simulink model "sampleModel7126_pp"  (R2018a)
settings: Solver=VariableStepAuto  StartTime=0.0  StopTime=10.0  RelTol=1e-3
undefined symbols (not defined in the file or in its folder): DiscIntNeverNeededParam
libraries: simulink x367
(part 3 of 8)

== system sampleModel7126_pp/cfblk260 ==
  cfblk1 : Inport
  cfblk9 : Inport  Port=2
  Action Port : ActionPort  ActionType=else
  cfblk13 : Delay
  cfblk3 : simulink/Discrete/Transfer Fcn Real Zero  ZeroZ=0.75  ICPrevInput=0.0  DoSatur=off
      settings: SourceProductName=Simulink  SourceProductBaseCode=SL
  cfblk4 : simulink/Continuous/PID Controller  Controller=PID  TimeDomain=Discrete-time  SampleTime=-1  IntegratorMethod=Forward Euler  FilterMethod=Forward Euler  Form=Parallel  UseFilter=on  ControllerParametersSource=internal  P=1  I=1  D=0  N=100  InitialConditionSource=internal  InitialConditionForIntegrator=0  InitialConditionForFilter=0  ExternalReset=none  LimitOutput=off  UpperSaturationLimit=inf  LowerSaturationLimit=-inf  LinearizeAsGain=off  AntiWindupMode=none  Kb=1  TrackingMode=off  Kt=1  PParamMin=[]  PParamMax=[]  IParamMin=[]  IParamMax=[]  DParamMin=[]  DParamMax=[]  NParamMin=[]  NParamMax=[]  KbParamMin=[]  KbParamMax=[]  KtParamMin=[]  KtParamMax=[]  POutMin=[]  POutMax=[]  IOutMin=[]  IOutMax=[]  DOutMin=[]  DOutMax=[]  NOutMin=[]  NOutMax=[]  KbOutMin=[]  KbOutMax=[]  KtOutMin=[]  KtOutMax=[]  IntegratorOutMin=[]  IntegratorOutMax=[]  FilterOutMin=[]  FilterOutMax=[]  SumOutMin=[]  SumOutMax=[]  SumI1OutMin=[]  SumI1OutMax=[]  SumI2OutMin=[]  SumI2OutMax=[]  SumI3OutMin=[]  SumI3OutMax=[]  SumDOutMin=[]  SumDOutMax=[]  SaturationOutMin=[]  SaturationOutMax=[]  IntegratorContinuousStateAttributes=''  IntegratorStateMustResolveToSignalObject=off  IntegratorRTWStateStorageClass=Auto  FilterContinuousStateAttributes=''  FilterStateMustResolveToSignalObject=off  FilterRTWStateStorageClass=Auto  DifferentiatorICPrevScaledInput=0  DifferentiatorOutMin=[]  DifferentiatorOutMax=[]  FilterDiffOutCoefMin=[]  FilterDiffOutCoefMax=[]  SumDenOutMin=[]  SumDenOutMax=[]  SumNumOutMin=[]  SumNumOutMax=[]  ReciprocalOutMin=[]  ReciprocalOutMax=[]  DivideOutMin=[]  DivideOutMax=[]  TunerSelectOption=Transfer Function Based (PID Tuner App)
  cfblk5 : DiscreteIntegrator  SampleTime=-1  OutDataTypeStr=double  ICPrevOutput=DiscIntNeverNeededParam  ICPrevScaledInput=DiscIntNeverNeededParam
  cfblk6 : Delay
  cfblk7 : Delay  DelayLengthSource=Input port
      settings: InputPortMap=u0,p1
  cfblk8 : simulink/Discrete/Transfer Fcn Lead or Lag  PoleZ=0.95  ZeroZ=0.75  ICPrevOutput=0.0  ICPrevInput=0.0  DoSatur=off
      settings: SourceProductName=Simulink  SourceProductBaseCode=SL
  cyemi_{449..456} (8 alike) : DataTypeConversion  OutDataTypeStr=double
  cfblk2 : Outport
  cfblk10 : Outport  Port=2
  cfblk11 : Outport  Port=3
  cfblk12 : Outport  Port=4
  wires:
  cfblk8/1 -> cfblk10/1
  cfblk4/1 -> cfblk12/1, cyemi_453/1
  cfblk3/1 -> cyemi_451/1, cyemi_452/1
  cfblk9/1 -> cfblk11/1, cfblk2/1
  cyemi_449/1 -> cfblk13/1
  cfblk5/1 -> cyemi_449/1
  cyemi_450/1 -> cfblk3/1
  cfblk13/1 -> cyemi_450/1
  cyemi_451/1 -> cfblk4/1
  cyemi_452/1 -> cfblk5/1
  cyemi_453/1 -> cfblk6/1
  cyemi_454/1 -> cfblk7/1
  cfblk6/1 -> cyemi_454/1
  cyemi_455/1 -> cfblk7/2
  cfblk1/1 -> cyemi_455/1
  cyemi_456/1 -> cfblk8/1
  cfblk7/1 -> cyemi_456/1

== system sampleModel7126_pp/cfblk261 ==
  cfblk1 : Inport
  Action Port : ActionPort  ActionType=then
  cfblk10 : simulink/Discrete/Difference  ICPrevInput=0.0  OutMin=[]  OutMax=[]  OutDataTypeStr=double  OutputDataTypeScalingMode=double  OutDataType=fixdt(1, 16)  OutScaling=2^-10  DoSatur=off
  cfblk11 : If  SampleTime=1
  cfblk13 : Subsystem  TreatAsAtomicUnit=on
  cfblk14 : Subsystem  TreatAsAtomicUnit=on
  cfblk15 : Delay
  cfblk16 : Delay
  cfblk17 : Delay
  cfblk3 : simulink/Discrete/Difference  ICPrevInput=0.0  OutMin=[]  OutMax=[]  OutDataTypeStr=double  OutputDataTypeScalingMode=double  OutDataType=fixdt(1, 16)  OutScaling=2^-10  DoSatur=off
  cfblk4 : DiscreteFilter
  cfblk5 : DiscreteTransferFcn
  cfblk6 : simulink/Continuous/PID Controller (2DOF)  Controller=PID  TimeDomain=Discrete-time  SampleTime=-1  IntegratorMethod=Forward Euler  FilterMethod=Forward Euler  Form=Parallel  UseFilter=on  ControllerParametersSource=internal  P=1  I=1  D=0  N=100  b=1  c=1  InitialConditionSource=internal  InitialConditionForIntegrator=0  InitialConditionForFilter=0  ExternalReset=none  LimitOutput=off  UpperSaturationLimit=inf  LowerSaturationLimit=-inf  LinearizeAsGain=off  AntiWindupMode=none  Kb=1  TrackingMode=off  Kt=1  PParamMin=[]  PParamMax=[]  IParamMin=[]  IParamMax=[]  DParamMin=[]  DParamMax=[]  NParamMin=[]  NParamMax=[]  bParamMin=[]  bParamMax=[]  cParamMin=[]  cParamMax=[]  KbParamMin=[]  KbParamMax=[]  KtParamMin=[]  KtParamMax=[]  POutMin=[]  POutMax=[]  IOutMin=[]  IOutMax=[]  DOutMin=[]  DOutMax=[]  NOutMin=[]  NOutMax=[]  bOutMin=[]  bOutMax=[]  cOutMin=[]  cOutMax=[]  KbOutMin=[]  KbOutMax=[]  KtOutMin=[]  KtOutMax=[]  IntegratorOutMin=[]  IntegratorOutMax=[]  FilterOutMin=[]  FilterOutMax=[]  SumOutMin=[]  SumOutMax=[]  Sum1OutMin=[]  Sum1OutMax=[]  Sum2OutMin=[]  Sum2OutMax=[]  Sum3OutMin=[]  Sum3OutMax=[]  SumI1OutMin=[]  SumI1OutMax=[]  SumI2OutMin=[]  SumI2OutMax=[]  SumI3OutMin=[]  SumI3OutMax=[]  SumDOutMin=[]  SumDOutMax=[]  SaturationOutMin=[]  SaturationOutMax=[]  IntegratorContinuousStateAttributes=''  IntegratorStateMustResolveToSignalObject=off  IntegratorRTWStateStorageClass=Auto  FilterContinuousStateAttributes=''  FilterStateMustResolveToSignalObject=off  FilterRTWStateStorageClass=Auto  DifferentiatorICPrevScaledInput=0  DifferentiatorOutMin=[]  DifferentiatorOutMax=[]  FilterDiffOutCoefMin=[]  FilterDiffOutCoefMax=[]  SumDenOutMin=[]  SumDenOutMax=[]  SumNumOutMin=[]  SumNumOutMax=[]  ReciprocalOutMin=[]  ReciprocalOutMax=[]  DivideOutMin=[]  DivideOutMax=[]  TunerSelectOption=Transfer Function Based (PID Tuner App)
  cfblk7 : Delay  ShowEnablePort=on
      settings: InputPortMap=u0,e6
  cfblk8 : DiscreteZeroPole  Poles=[0 0.5]  Gain=1  SampleTime=-1
  cfblk9 : simulink/Continuous/PID Controller  Controller=PID  TimeDomain=Discrete-time  SampleTime=-1  IntegratorMethod=Forward Euler  FilterMethod=Forward Euler  Form=Parallel  UseFilter=on  ControllerParametersSource=internal  P=1  I=1  D=0  N=100  InitialConditionSource=internal  InitialConditionForIntegrator=0  InitialConditionForFilter=0  ExternalReset=none  LimitOutput=off  UpperSaturationLimit=inf  LowerSaturationLimit=-inf  LinearizeAsGain=off  AntiWindupMode=none  Kb=1  TrackingMode=off  Kt=1  PParamMin=[]  PParamMax=[]  IParamMin=[]  IParamMax=[]  DParamMin=[]  DParamMax=[]  NParamMin=[]  NParamMax=[]  KbParamMin=[]  KbParamMax=[]  KtParamMin=[]  KtParamMax=[]  POutMin=[]  POutMax=[]  IOutMin=[]  IOutMax=[]  DOutMin=[]  DOutMax=[]  NOutMin=[]  NOutMax=[]  KbOutMin=[]  KbOutMax=[]  KtOutMin=[]  KtOutMax=[]  IntegratorOutMin=[]  IntegratorOutMax=[]  FilterOutMin=[]  FilterOutMax=[]  SumOutMin=[]  SumOutMax=[]  SumI1OutMin=[]  SumI1OutMax=[]  SumI2OutMin=[]  SumI2OutMax=[]  SumI3OutMin=[]  SumI3OutMax=[]  SumDOutMin=[]  SumDOutMax=[]  SaturationOutMin=[]  SaturationOutMax=[]  IntegratorContinuousStateAttributes=''  IntegratorStateMustResolveToSignalObject=off  IntegratorRTWStateStorageClass=Auto  FilterContinuousStateAttributes=''  FilterStateMustResolveToSignalObject=off  FilterRTWStateStorageClass=Auto  DifferentiatorICPrevScaledInput=0  DifferentiatorOutMin=[]  DifferentiatorOutMax=[]  FilterDiffOutCoefMin=[]  FilterDiffOutCoefMax=[]  SumDenOutMin=[]  SumDenOutMax=[]  SumNumOutMin=[]  SumNumOutMax=[]  ReciprocalOutMin=[]  ReciprocalOutMax=[]  DivideOutMin=[]  DivideOutMax=[]  TunerSelectOption=Transfer Function Based (PID Tuner App)
  cyemi_{458..460,469..470,473..484} (17 alike) : DataTypeConversion  OutDataTypeStr=double
  cfblk2 : Outport
  cfblk12 : Outport  Port=2
  wires:
  cfblk7/1 -> cyemi_459/1, cyemi_476/1
  cfblk9/1 -> cfblk2/1
  cfblk8/1 -> cyemi_473/1, cyemi_478/1
  cfblk13/1(cfblk2) -> cyemi_470/1, cyemi_479/1
  cfblk14/1(cfblk2) -> cfblk12/1
  cfblk11/1 -> cfblk13/Action
  cfblk11/2 -> cfblk14/Action
  cyemi_458/1 -> cfblk10/1
  cfblk14/3(cfblk7) -> cyemi_458/1
  cyemi_459/1 -> cfblk11/1
  cyemi_460/1 -> cfblk13/1(cfblk1)
  cfblk3/1 -> cyemi_460/1
  cyemi_469/1 -> cfblk14/1(cfblk1)
  cfblk16/1 -> cyemi_469/1
  cyemi_470/1 -> cfblk14/2(cfblk5)
  cyemi_473/1 -> cfblk15/1
  cyemi_474/1 -> cfblk16/1
  cfblk4/1 -> cyemi_474/1
  cyemi_475/1 -> cfblk17/1
  cfblk10/1 -> cyemi_475/1
  cyemi_476/1 -> cfblk3/1
  cyemi_477/1 -> cfblk4/1
  cfblk14/2(cfblk6) -> cyemi_477/1
  cyemi_478/1 -> cfblk5/1
  cyemi_479/1 -> cfblk6/1
  cyemi_480/1 -> cfblk6/2
  cfblk15/1 -> cyemi_480/1
  cyemi_481/1 -> cfblk7/1
  cfblk1/1 -> cyemi_481/1
  cyemi_482/1 -> cfblk7/2
  cfblk17/1 -> cyemi_482/1
  cyemi_483/1 -> cfblk8/1
  cfblk6/1 -> cyemi_483/1
  cyemi_484/1 -> cfblk9/1
  cfblk5/1 -> cyemi_484/1

== system sampleModel7126_pp/cfblk262 ==
  cfblk1 : Inport
  cfblk9 : Inport  Port=2
  Action Port : ActionPort  ActionType=else
  cfblk11 : Delay
  cfblk3 : simulink/Continuous/PID Controller  Controller=PID  TimeDomain=Discrete-time  SampleTime=-1  IntegratorMethod=Forward Euler  FilterMethod=Forward Euler  Form=Parallel  UseFilter=on  ControllerParametersSource=internal  P=1  I=1  D=0  N=100  InitialConditionSource=internal  InitialConditionForIntegrator=0  InitialConditionForFilter=0  ExternalReset=none  LimitOutput=off  UpperSaturationLimit=inf  LowerSaturationLimit=-inf  LinearizeAsGain=off  AntiWindupMode=none  Kb=1  TrackingMode=off  Kt=1  PParamMin=[]  PParamMax=[]  IParamMin=[]  IParamMax=[]  DParamMin=[]  DParamMax=[]  NParamMin=[]  NParamMax=[]  KbParamMin=[]  KbParamMax=[]  KtParamMin=[]  KtParamMax=[]  POutMin=[]  POutMax=[]  IOutMin=[]  IOutMax=[]  DOutMin=[]  DOutMax=[]  NOutMin=[]  NOutMax=[]  KbOutMin=[]  KbOutMax=[]  KtOutMin=[]  KtOutMax=[]  IntegratorOutMin=[]  IntegratorOutMax=[]  FilterOutMin=[]  FilterOutMax=[]  SumOutMin=[]  SumOutMax=[]  SumI1OutMin=[]  SumI1OutMax=[]  SumI2OutMin=[]  SumI2OutMax=[]  SumI3OutMin=[]  SumI3OutMax=[]  SumDOutMin=[]  SumDOutMax=[]  SaturationOutMin=[]  SaturationOutMax=[]  IntegratorContinuousStateAttributes=''  IntegratorStateMustResolveToSignalObject=off  IntegratorRTWStateStorageClass=Auto  FilterContinuousStateAttributes=''  FilterStateMustResolveToSignalObject=off  FilterRTWStateStorageClass=Auto  DifferentiatorICPrevScaledInput=0  DifferentiatorOutMin=[]  DifferentiatorOutMax=[]  FilterDiffOutCoefMin=[]  FilterDiffOutCoefMax=[]  SumDenOutMin=[]  SumDenOutMax=[]  SumNumOutMin=[]  SumNumOutMax=[]  ReciprocalOutMin=[]  ReciprocalOutMax=[]  DivideOutMin=[]  DivideOutMax=[]  TunerSelectOption=Transfer Function Based (PID Tuner App)
  cfblk4 : DiscreteIntegrator  SampleTime=-1  OutDataTypeStr=double  ICPrevOutput=DiscIntNeverNeededParam  ICPrevScaledInput=DiscIntNeverNeededParam
  cfblk5 : Delay  DelayLengthSource=Input port
      settings: InputPortMap=u0,p1
  cfblk6 : simulink/Discrete/Transfer Fcn Real Zero  ZeroZ=0.75  ICPrevInput=0.0  DoSatur=off
      settings: SourceProductName=Simulink  SourceProductBaseCode=SL
  cfblk7 : DiscreteFilter
  cfblk8 : Delay
  cyemi_{487..494} (8 alike) : DataTypeConversion  OutDataTypeStr=double
  cfblk2 : Outport
  cfblk10 : Outport  Port=2
  wires:
  cfblk7/1 -> cfblk2/1
  cfblk9/1 -> cfblk10/1
  cfblk8/1 -> cyemi_487/1, cyemi_488/1
  cyemi_487/1 -> cfblk11/1
  cyemi_488/1 -> cfblk3/1
  cyemi_489/1 -> cfblk4/1
  cfblk1/1 -> cyemi_489/1
  cyemi_490/1 -> cfblk5/1
  cfblk6/1 -> cyemi_490/1
  cyemi_491/1 -> cfblk5/2
  cfblk11/1 -> cyemi_491/1
  cyemi_492/1 -> cfblk6/1
  cfblk4/1 -> cyemi_492/1
  cyemi_493/1 -> cfblk7/1
  cfblk3/1 -> cyemi_493/1
  cyemi_494/1 -> cfblk8/1
  cfblk5/1 -> cyemi_494/1

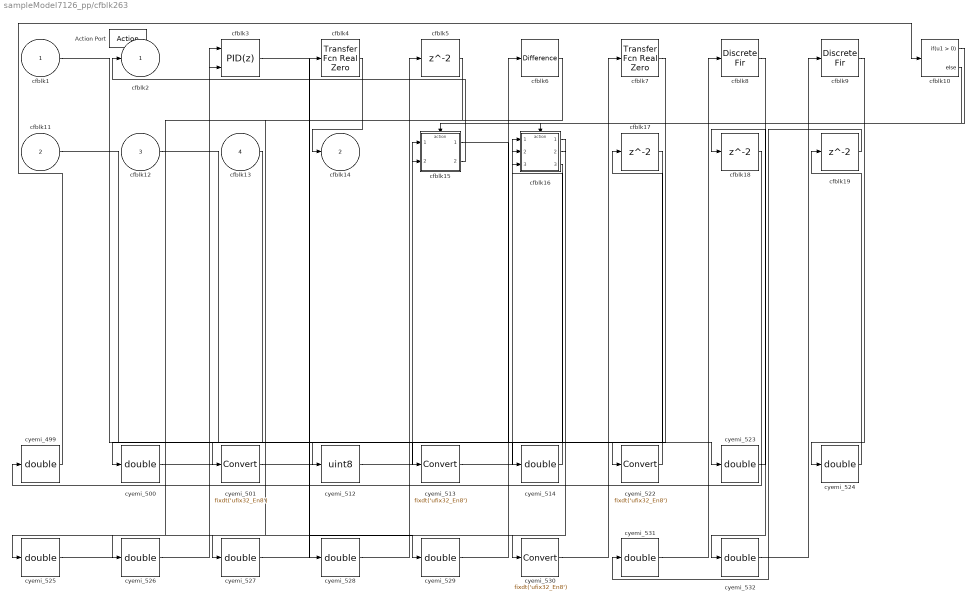
== system sampleModel7126_pp/cfblk263 ==
  cfblk1 : Inport
  cfblk11 : Inport  Port=2
  cfblk12 : Inport  Port=3
  cfblk13 : Inport  Port=4
  Action Port : ActionPort  ActionType=then
  cfblk10 : If  SampleTime=1
  cfblk15 : Subsystem  TreatAsAtomicUnit=on
  cfblk16 : Subsystem  TreatAsAtomicUnit=on
  cfblk{5,17..19} (4 alike) : Delay
  cfblk3 : simulink/Continuous/PID Controller (2DOF)  Controller=PID  TimeDomain=Discrete-time  SampleTime=-1  IntegratorMethod=Forward Euler  FilterMethod=Forward Euler  Form=Parallel  UseFilter=on  ControllerParametersSource=internal  P=1  I=1  D=0  N=100  b=1  c=1  InitialConditionSource=internal  InitialConditionForIntegrator=0  InitialConditionForFilter=0  ExternalReset=none  LimitOutput=off  UpperSaturationLimit=inf  LowerSaturationLimit=-inf  LinearizeAsGain=off  AntiWindupMode=none  Kb=1  TrackingMode=off  Kt=1  PParamMin=[]  PParamMax=[]  IParamMin=[]  IParamMax=[]  DParamMin=[]  DParamMax=[]  NParamMin=[]  NParamMax=[]  bParamMin=[]  bParamMax=[]  cParamMin=[]  cParamMax=[]  KbParamMin=[]  KbParamMax=[]  KtParamMin=[]  KtParamMax=[]  POutMin=[]  POutMax=[]  IOutMin=[]  IOutMax=[]  DOutMin=[]  DOutMax=[]  NOutMin=[]  NOutMax=[]  bOutMin=[]  bOutMax=[]  cOutMin=[]  cOutMax=[]  KbOutMin=[]  KbOutMax=[]  KtOutMin=[]  KtOutMax=[]  IntegratorOutMin=[]  IntegratorOutMax=[]  FilterOutMin=[]  FilterOutMax=[]  SumOutMin=[]  SumOutMax=[]  Sum1OutMin=[]  Sum1OutMax=[]  Sum2OutMin=[]  Sum2OutMax=[]  Sum3OutMin=[]  Sum3OutMax=[]  SumI1OutMin=[]  SumI1OutMax=[]  SumI2OutMin=[]  SumI2OutMax=[]  SumI3OutMin=[]  SumI3OutMax=[]  SumDOutMin=[]  SumDOutMax=[]  SaturationOutMin=[]  SaturationOutMax=[]  IntegratorContinuousStateAttributes=''  IntegratorStateMustResolveToSignalObject=off  IntegratorRTWStateStorageClass=Auto  FilterContinuousStateAttributes=''  FilterStateMustResolveToSignalObject=off  FilterRTWStateStorageClass=Auto  DifferentiatorICPrevScaledInput=0  DifferentiatorOutMin=[]  DifferentiatorOutMax=[]  FilterDiffOutCoefMin=[]  FilterDiffOutCoefMax=[]  SumDenOutMin=[]  SumDenOutMax=[]  SumNumOutMin=[]  SumNumOutMax=[]  ReciprocalOutMin=[]  ReciprocalOutMax=[]  DivideOutMin=[]  DivideOutMax=[]  TunerSelectOption=Transfer Function Based (PID Tuner App)
  cfblk4 : simulink/Discrete/Transfer Fcn Real Zero  ZeroZ=0.75  ICPrevInput=0.0  DoSatur=off
      settings: SourceProductName=Simulink  SourceProductBaseCode=SL
  cfblk6 : simulink/Discrete/Difference  ICPrevInput=0.0  OutMin=[]  OutMax=[]  OutDataTypeStr=double  OutputDataTypeScalingMode=double  OutDataType=fixdt(1, 16)  OutScaling=2^-10  DoSatur=off
  cfblk7 : simulink/Discrete/Transfer Fcn Real Zero  ZeroZ=0.75  ICPrevInput=0.0  DoSatur=off
      settings: SourceProductName=Simulink  SourceProductBaseCode=SL
  cfblk8 : DiscreteFir
  cfblk9 : DiscreteFir
  cyemi_{499..500,514,523..529,531..532} (12 alike) : DataTypeConversion  OutDataTypeStr=double
  cyemi_{501,513,522,530} (4 alike) : DataTypeConversion  OutDataTypeStr=fixdt('ufix32_En8')
  cyemi_512 : DataTypeConversion  OutDataTypeStr=uint8
  cfblk2 : Outport
  cfblk14 : Outport  Port=2
  wires:
  cfblk4/1 -> cfblk14/1
  cfblk15/2(cfblk12) -> cfblk2/1
  cfblk10/1 -> cfblk15/Action
  cfblk10/2 -> cfblk16/Action
  cyemi_499/1 -> cfblk10/1
  cfblk18/1 -> cyemi_499/1
  cyemi_500/1 -> cfblk15/1(cfblk1)
  cfblk13/1 -> cyemi_500/1
  cyemi_501/1 -> cfblk15/2(cfblk11)
  cfblk16/3(cfblk13) -> cyemi_501/1
  cyemi_512/1 -> cfblk16/1(cfblk1)
  cfblk1/1 -> cyemi_512/1
  cyemi_513/1 -> cfblk16/2(cfblk10)
  cfblk17/1 -> cyemi_513/1
  cyemi_514/1 -> cfblk16/3(cfblk11)
  cfblk11/1 -> cyemi_514/1
  cyemi_522/1 -> cfblk17/1
  cfblk7/1 -> cyemi_522/1
  cyemi_523/1 -> cfblk18/1
  cfblk15/1(cfblk2) -> cyemi_523/1
  cyemi_524/1 -> cfblk19/1
  cfblk9/1 -> cyemi_524/1
  cyemi_525/1 -> cfblk3/1
  cfblk16/1(cfblk2) -> cyemi_525/1
  cyemi_526/1 -> cfblk3/2
  cfblk5/1 -> cyemi_526/1
  cyemi_527/1 -> cfblk4/1
  cfblk6/1 -> cyemi_527/1
  cyemi_528/1 -> cfblk5/1
  cfblk12/1 -> cyemi_528/1
  cyemi_529/1 -> cfblk6/1
  cfblk3/1 -> cyemi_529/1
  cyemi_530/1 -> cfblk7/1
  cfblk16/2(cfblk12) -> cyemi_530/1
  cyemi_531/1 -> cfblk8/1
  cfblk19/1 -> cyemi_531/1
  cyemi_532/1 -> cfblk9/1
  cfblk8/1 -> cyemi_532/1

== system sampleModel7126_pp/cfblk264 ==
  cfblk1 : Inport
  cfblk12 : Inport  Port=2
  Action Port : ActionPort  ActionType=else
  cfblk10 : simulink/Discrete/Difference  ICPrevInput=0.0  OutMin=[]  OutMax=[]  OutDataTypeStr=double  OutputDataTypeScalingMode=double  OutDataType=fixdt(1, 16)  OutScaling=2^-10  DoSatur=off
  cfblk11 : Delay  DelayLengthSource=Input port
      settings: InputPortMap=u0,p1
  cfblk15 : Delay
  cfblk16 : Delay
  cfblk3 : DiscreteFir
  cfblk4 : DiscreteZeroPole  Poles=[0 0.5]  Gain=1  SampleTime=-1
  cfblk5 : DiscreteFir
  cfblk6 : DiscreteTransferFcn
  cfblk7 : Delay  DelayLengthSource=Input port
      settings: InputPortMap=u0,p1
  cfblk8 : DiscreteTransferFcn
  cfblk9 : simulink/Continuous/PID Controller  Controller=PID  TimeDomain=Discrete-time  SampleTime=-1  IntegratorMethod=Forward Euler  FilterMethod=Forward Euler  Form=Parallel  UseFilter=on  ControllerParametersSource=internal  P=1  I=1  D=0  N=100  InitialConditionSource=internal  InitialConditionForIntegrator=0  InitialConditionForFilter=0  ExternalReset=none  LimitOutput=off  UpperSaturationLimit=inf  LowerSaturationLimit=-inf  LinearizeAsGain=off  AntiWindupMode=none  Kb=1  TrackingMode=off  Kt=1  PParamMin=[]  PParamMax=[]  IParamMin=[]  IParamMax=[]  DParamMin=[]  DParamMax=[]  NParamMin=[]  NParamMax=[]  KbParamMin=[]  KbParamMax=[]  KtParamMin=[]  KtParamMax=[]  POutMin=[]  POutMax=[]  IOutMin=[]  IOutMax=[]  DOutMin=[]  DOutMax=[]  NOutMin=[]  NOutMax=[]  KbOutMin=[]  KbOutMax=[]  KtOutMin=[]  KtOutMax=[]  IntegratorOutMin=[]  IntegratorOutMax=[]  FilterOutMin=[]  FilterOutMax=[]  SumOutMin=[]  SumOutMax=[]  SumI1OutMin=[]  SumI1OutMax=[]  SumI2OutMin=[]  SumI2OutMax=[]  SumI3OutMin=[]  SumI3OutMax=[]  SumDOutMin=[]  SumDOutMax=[]  SaturationOutMin=[]  SaturationOutMax=[]  IntegratorContinuousStateAttributes=''  IntegratorStateMustResolveToSignalObject=off  IntegratorRTWStateStorageClass=Auto  FilterContinuousStateAttributes=''  FilterStateMustResolveToSignalObject=off  FilterRTWStateStorageClass=Auto  DifferentiatorICPrevScaledInput=0  DifferentiatorOutMin=[]  DifferentiatorOutMax=[]  FilterDiffOutCoefMin=[]  FilterDiffOutCoefMax=[]  SumDenOutMin=[]  SumDenOutMax=[]  SumNumOutMin=[]  SumNumOutMax=[]  ReciprocalOutMin=[]  ReciprocalOutMax=[]  DivideOutMin=[]  DivideOutMax=[]  TunerSelectOption=Transfer Function Based (PID Tuner App)
  cyemi_{535..547} (13 alike) : DataTypeConversion  OutDataTypeStr=double
  cfblk2 : Outport
  cfblk13 : Outport  Port=2
  cfblk14 : Outport  Port=3
  wires:
  cfblk9/1 -> cfblk14/1, cyemi_537/1
  cfblk6/1 -> cfblk2/1, cyemi_538/1
  cfblk11/1 -> cfblk13/1
  cfblk10/1 -> cyemi_539/1, cyemi_541/1
  cyemi_535/1 -> cfblk10/1
  cfblk8/1 -> cyemi_535/1
  cyemi_536/1 -> cfblk11/1
  cfblk12/1 -> cyemi_536/1
  cyemi_537/1 -> cfblk11/2
  cyemi_538/1 -> cfblk15/1
  cyemi_539/1 -> cfblk16/1
  cyemi_540/1 -> cfblk3/1
  cfblk4/1 -> cyemi_540/1
  cyemi_541/1 -> cfblk4/1
  cyemi_542/1 -> cfblk5/1
  cfblk7/1 -> cyemi_542/1
  cyemi_543/1 -> cfblk6/1
  cfblk5/1 -> cyemi_543/1
  cyemi_544/1 -> cfblk7/1
  cfblk3/1 -> cyemi_544/1
  cyemi_545/1 -> cfblk7/2
  cfblk15/1 -> cyemi_545/1
  cyemi_546/1 -> cfblk8/1
  cfblk16/1 -> cyemi_546/1
  cyemi_547/1 -> cfblk9/1
  cfblk1/1 -> cyemi_547/1

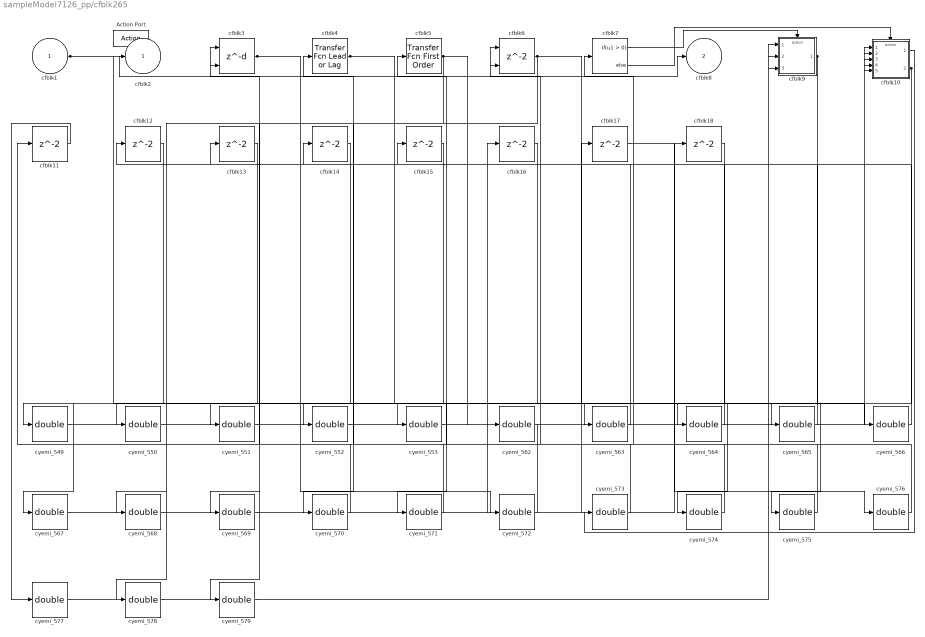
== system sampleModel7126_pp/cfblk265 ==
  cfblk1 : Inport
  Action Port : ActionPort  ActionType=then
  cfblk10 : Subsystem  TreatAsAtomicUnit=on
  cfblk{11..18} (8 alike) : Delay
  cfblk3 : Delay  DelayLengthSource=Input port
      settings: InputPortMap=u0,p1
  cfblk4 : simulink/Discrete/Transfer Fcn Lead or Lag  PoleZ=0.95  ZeroZ=0.75  ICPrevOutput=0.0  ICPrevInput=0.0  DoSatur=off
      settings: SourceProductName=Simulink  SourceProductBaseCode=SL
  cfblk5 : simulink/Discrete/Transfer Fcn First Order  PoleZ=0.95  ICPrevOutput=0.0  DoSatur=off
      settings: SourceProductName=Simulink
  cfblk6 : Delay  ShowEnablePort=on
      settings: InputPortMap=u0,e6
  cfblk7 : If  SampleTime=1
  cfblk9 : Subsystem  TreatAsAtomicUnit=on
  cyemi_{549..553,562..579} (23 alike) : DataTypeConversion  OutDataTypeStr=double
  cfblk2 : Outport
  cfblk8 : Outport  Port=2
  wires:
  cfblk1/1 -> cfblk8/1, cfblk2/1, cyemi_553/1
  cfblk6/1 -> cyemi_566/1, cyemi_570/1
  cfblk10/2(cfblk15) -> cyemi_571/1, cyemi_575/1
  cfblk3/1 -> cyemi_565/1, cyemi_572/1
  cfblk5/1 -> cyemi_562/1, cyemi_568/1, cyemi_569/1
  cfblk4/1 -> cyemi_563/1, cyemi_564/1
  cfblk9/1(cfblk2) -> cyemi_567/1, cyemi_574/1
  cfblk7/1 -> cfblk9/Action
  cfblk7/2 -> cfblk10/Action
  cyemi_549/1 -> cfblk10/1(cfblk1)
  cfblk12/1 -> cyemi_549/1
  cyemi_550/1 -> cfblk10/2(cfblk11)
  cfblk18/1 -> cyemi_550/1
  cyemi_551/1 -> cfblk10/3(cfblk12)
  cfblk14/1 -> cyemi_551/1
  cyemi_552/1 -> cfblk10/4(cfblk13)
  cfblk16/1 -> cyemi_552/1
  cyemi_553/1 -> cfblk10/5(cfblk14)
  cyemi_562/1 -> cfblk11/1
  cyemi_563/1 -> cfblk12/1
  cyemi_564/1 -> cfblk13/1
  cyemi_565/1 -> cfblk14/1
  cyemi_566/1 -> cfblk15/1
  cyemi_567/1 -> cfblk16/1
  cyemi_568/1 -> cfblk17/1
  cyemi_569/1 -> cfblk18/1
  cyemi_570/1 -> cfblk3/1
  cyemi_571/1 -> cfblk3/2
  cyemi_572/1 -> cfblk4/1
  cyemi_573/1 -> cfblk5/1
  cfblk10/1(cfblk2) -> cyemi_573/1
  cyemi_574/1 -> cfblk6/1
  cyemi_575/1 -> cfblk6/2
  cyemi_576/1 -> cfblk7/1
  cfblk17/1 -> cyemi_576/1
  cyemi_577/1 -> cfblk9/1(cfblk1)
  cfblk11/1 -> cyemi_577/1
  cyemi_578/1 -> cfblk9/2(cfblk10)
  cfblk13/1 -> cyemi_578/1
  cyemi_579/1 -> cfblk9/3(cfblk11)
  cfblk15/1 -> cyemi_579/1

== system sampleModel7126_pp/cfblk266 ==
  cfblk1 : Inport
  Action Port : ActionPort  ActionType=else
  cfblk10 : Subsystem  TreatAsAtomicUnit=on
  cfblk{11..14} (4 alike) : Delay
  cfblk3 : UnitDelay  SampleTime=-1
  cfblk4 : DiscreteIntegrator  SampleTime=-1  OutDataTypeStr=double  ICPrevOutput=DiscIntNeverNeededParam  ICPrevScaledInput=DiscIntNeverNeededParam
  cfblk5 : DiscreteTransferFcn
  cfblk6 : simulink/Continuous/PID Controller (2DOF)  Controller=PID  TimeDomain=Discrete-time  SampleTime=-1  IntegratorMethod=Forward Euler  FilterMethod=Forward Euler  Form=Parallel  UseFilter=on  ControllerParametersSource=internal  P=1  I=1  D=0  N=100  b=1  c=1  InitialConditionSource=internal  InitialConditionForIntegrator=0  InitialConditionForFilter=0  ExternalReset=none  LimitOutput=off  UpperSaturationLimit=inf  LowerSaturationLimit=-inf  LinearizeAsGain=off  AntiWindupMode=none  Kb=1  TrackingMode=off  Kt=1  PParamMin=[]  PParamMax=[]  IParamMin=[]  IParamMax=[]  DParamMin=[]  DParamMax=[]  NParamMin=[]  NParamMax=[]  bParamMin=[]  bParamMax=[]  cParamMin=[]  cParamMax=[]  KbParamMin=[]  KbParamMax=[]  KtParamMin=[]  KtParamMax=[]  POutMin=[]  POutMax=[]  IOutMin=[]  IOutMax=[]  DOutMin=[]  DOutMax=[]  NOutMin=[]  NOutMax=[]  bOutMin=[]  bOutMax=[]  cOutMin=[]  cOutMax=[]  KbOutMin=[]  KbOutMax=[]  KtOutMin=[]  KtOutMax=[]  IntegratorOutMin=[]  IntegratorOutMax=[]  FilterOutMin=[]  FilterOutMax=[]  SumOutMin=[]  SumOutMax=[]  Sum1OutMin=[]  Sum1OutMax=[]  Sum2OutMin=[]  Sum2OutMax=[]  Sum3OutMin=[]  Sum3OutMax=[]  SumI1OutMin=[]  SumI1OutMax=[]  SumI2OutMin=[]  SumI2OutMax=[]  SumI3OutMin=[]  SumI3OutMax=[]  SumDOutMin=[]  SumDOutMax=[]  SaturationOutMin=[]  SaturationOutMax=[]  IntegratorContinuousStateAttributes=''  IntegratorStateMustResolveToSignalObject=off  IntegratorRTWStateStorageClass=Auto  FilterContinuousStateAttributes=''  FilterStateMustResolveToSignalObject=off  FilterRTWStateStorageClass=Auto  DifferentiatorICPrevScaledInput=0  DifferentiatorOutMin=[]  DifferentiatorOutMax=[]  FilterDiffOutCoefMin=[]  FilterDiffOutCoefMax=[]  SumDenOutMin=[]  SumDenOutMax=[]  SumNumOutMin=[]  SumNumOutMax=[]  ReciprocalOutMin=[]  ReciprocalOutMax=[]  DivideOutMin=[]  DivideOutMax=[]  TunerSelectOption=Transfer Function Based (PID Tuner App)
  cfblk7 : DiscreteFilter
  cfblk8 : If  SampleTime=1
  cfblk9 : Subsystem  TreatAsAtomicUnit=on
  cyemi_{590,598..611} (15 alike) : DataTypeConversion  OutDataTypeStr=double
  cfblk2 : Outport
  wires:
  cfblk10/2(cfblk7) -> cfblk2/1
  cfblk4/1 -> cyemi_599/1, cyemi_600/1
  cfblk5/1 -> cyemi_590/1, cyemi_610/1
  cfblk8/1 -> cfblk9/Action
  cfblk8/2 -> cfblk10/Action
  cyemi_590/1 -> cfblk10/1(cfblk1)
  cyemi_598/1 -> cfblk11/1
  cfblk9/1(cfblk2) -> cyemi_598/1
  cyemi_599/1 -> cfblk12/1
  cyemi_600/1 -> cfblk13/1
  cyemi_601/1 -> cfblk14/1
  cfblk7/1 -> cyemi_601/1
  cyemi_602/1 -> cfblk3/1
  cfblk1/1 -> cyemi_602/1
  cyemi_603/1 -> cfblk4/1
  cfblk9/2(cfblk8) -> cyemi_603/1
  cyemi_604/1 -> cfblk5/1
  cfblk3/1 -> cyemi_604/1
  cyemi_605/1 -> cfblk6/1
  cfblk11/1 -> cyemi_605/1
  cyemi_606/1 -> cfblk6/2
  cfblk10/1(cfblk2) -> cyemi_606/1
  cyemi_607/1 -> cfblk7/1
  cfblk6/1 -> cyemi_607/1
  cyemi_608/1 -> cfblk8/1
  cfblk14/1 -> cyemi_608/1
  cyemi_609/1 -> cfblk9/1(cfblk1)
  cfblk12/1 -> cyemi_609/1
  cyemi_610/1 -> cfblk9/2(cfblk6)
  cyemi_611/1 -> cfblk9/3(cfblk7)
  cfblk13/1 -> cyemi_611/1

== system sampleModel7126_pp/cfblk267 ==
  cfblk1 : Inport
  cfblk13 : Inport  Port=2
  Action Port : ActionPort  ActionType=then
  cfblk10 : DiscreteFilter
  cfblk11 : Delay
  cfblk12 : simulink/Discrete/Transfer Fcn Real Zero  ZeroZ=0.75  ICPrevInput=0.0  DoSatur=off
      settings: SourceProductName=Simulink  SourceProductBaseCode=SL
  cfblk16 : DataTypeConversion  OutDataTypeStr=double
  cfblk3 : DiscreteFir
  cfblk4 : UnitDelay  SampleTime=-1
  cfblk5 : simulink/Continuous/PID Controller  Controller=PID  TimeDomain=Discrete-time  SampleTime=-1  IntegratorMethod=Forward Euler  FilterMethod=Forward Euler  Form=Parallel  UseFilter=on  ControllerParametersSource=internal  P=1  I=1  D=0  N=100  InitialConditionSource=internal  InitialConditionForIntegrator=0  InitialConditionForFilter=0  ExternalReset=none  LimitOutput=off  UpperSaturationLimit=inf  LowerSaturationLimit=-inf  LinearizeAsGain=off  AntiWindupMode=none  Kb=1  TrackingMode=off  Kt=1  PParamMin=[]  PParamMax=[]  IParamMin=[]  IParamMax=[]  DParamMin=[]  DParamMax=[]  NParamMin=[]  NParamMax=[]  KbParamMin=[]  KbParamMax=[]  KtParamMin=[]  KtParamMax=[]  POutMin=[]  POutMax=[]  IOutMin=[]  IOutMax=[]  DOutMin=[]  DOutMax=[]  NOutMin=[]  NOutMax=[]  KbOutMin=[]  KbOutMax=[]  KtOutMin=[]  KtOutMax=[]  IntegratorOutMin=[]  IntegratorOutMax=[]  FilterOutMin=[]  FilterOutMax=[]  SumOutMin=[]  SumOutMax=[]  SumI1OutMin=[]  SumI1OutMax=[]  SumI2OutMin=[]  SumI2OutMax=[]  SumI3OutMin=[]  SumI3OutMax=[]  SumDOutMin=[]  SumDOutMax=[]  SaturationOutMin=[]  SaturationOutMax=[]  IntegratorContinuousStateAttributes=''  IntegratorStateMustResolveToSignalObject=off  IntegratorRTWStateStorageClass=Auto  FilterContinuousStateAttributes=''  FilterStateMustResolveToSignalObject=off  FilterRTWStateStorageClass=Auto  DifferentiatorICPrevScaledInput=0  DifferentiatorOutMin=[]  DifferentiatorOutMax=[]  FilterDiffOutCoefMin=[]  FilterDiffOutCoefMax=[]  SumDenOutMin=[]  SumDenOutMax=[]  SumNumOutMin=[]  SumNumOutMax=[]  ReciprocalOutMin=[]  ReciprocalOutMax=[]  DivideOutMin=[]  DivideOutMax=[]  TunerSelectOption=Transfer Function Based (PID Tuner App)
  cfblk6 : simulink/Discrete/Transfer Fcn Real Zero  ZeroZ=0.75  ICPrevInput=0.0  DoSatur=off
      settings: SourceProductName=Simulink  SourceProductBaseCode=SL
  cfblk7 : DiscreteStateSpace  SampleTime=-1
  cfblk8 : DiscreteZeroPole  Poles=[0 0.5]  Gain=1  SampleTime=-1
  cfblk9 : Delay  ShowEnablePort=on
      settings: InputPortMap=u0,e6
  cyemi_{617..619,621..628} (11 alike) : DataTypeConversion  OutDataTypeStr=double
  cyemi_620 : DataTypeConversion  OutDataTypeStr=uint16
  cfblk2 : Outport
  cfblk14 : Outport  Port=2
  cfblk15 : Outport  Port=3
  wires:
  cfblk10/1 -> cfblk2/1
  cfblk4/1 -> cfblk14/1, cyemi_621/1
  cfblk7/1 -> cfblk15/1, cyemi_619/1
  cyemi_617/1 -> cfblk10/1
  cfblk9/1 -> cyemi_617/1
  cyemi_618/1 -> cfblk11/1
  cfblk8/1 -> cyemi_618/1
  cyemi_619/1 -> cfblk12/1
  cyemi_620/1 -> cfblk16/1
  cfblk13/1 -> cyemi_620/1
  cyemi_621/1 -> cfblk3/1
  cyemi_622/1 -> cfblk4/1
  cfblk6/1 -> cyemi_622/1
  cyemi_623/1 -> cfblk5/1
  cfblk12/1 -> cyemi_623/1
  cyemi_624/1 -> cfblk6/1
  cfblk1/1 -> cyemi_624/1
  cyemi_625/1 -> cfblk7/1
  cfblk3/1 -> cyemi_625/1
  cyemi_626/1 -> cfblk8/1
  cfblk16/1 -> cyemi_626/1
  cyemi_627/1 -> cfblk9/1
  cfblk5/1 -> cyemi_627/1
  cyemi_628/1 -> cfblk9/2
  cfblk11/1 -> cyemi_628/1

== system sampleModel7126_pp/cfblk268 ==
  cfblk1 : Inport
  cfblk9 : Inport  Port=2
  cfblk10 : Inport  Port=3
  cfblk11 : Inport  Port=4
  Action Port : ActionPort  ActionType=else
  cfblk3 : DiscreteStateSpace  SampleTime=-1
  cfblk4 : DiscreteIntegrator  SampleTime=-1  OutDataTypeStr=double  ICPrevOutput=DiscIntNeverNeededParam  ICPrevScaledInput=DiscIntNeverNeededParam
  cfblk5 : simulink/Discrete/Transfer Fcn Real Zero  ZeroZ=0.75  ICPrevInput=0.0  DoSatur=off
      settings: SourceProductName=Simulink  SourceProductBaseCode=SL
  cfblk6 : DiscreteFir
  cfblk7 : Delay
  cfblk8 : simulink/Discrete/Transfer Fcn Lead or Lag  PoleZ=0.95  ZeroZ=0.75  ICPrevOutput=0.0  ICPrevInput=0.0  DoSatur=off
      settings: SourceProductName=Simulink  SourceProductBaseCode=SL
  cyemi_{633..638} (6 alike) : DataTypeConversion  OutDataTypeStr=double
  cfblk2 : Outport
  cfblk12 : Outport  Port=2
  cfblk13 : Outport  Port=3
  wires:
  cfblk8/1 -> cfblk12/1
  cfblk3/1 -> cfblk2/1
  cfblk4/1 -> cfblk13/1
  cyemi_633/1 -> cfblk3/1
  cfblk6/1 -> cyemi_633/1
  cyemi_634/1 -> cfblk4/1
  cfblk5/1 -> cyemi_634/1
  cyemi_635/1 -> cfblk5/1
  cfblk10/1 -> cyemi_635/1
  cyemi_636/1 -> cfblk6/1
  cfblk7/1 -> cyemi_636/1
  cyemi_637/1 -> cfblk7/1
  cfblk1/1 -> cyemi_637/1
  cyemi_638/1 -> cfblk8/1
  cfblk9/1 -> cyemi_638/1

== system sampleModel7126_pp/cfblk269 ==
  cfblk1 : Inport
  cfblk6 : Inport  Port=2
  Action Port : ActionPort  ActionType=then
  cfblk{10..14} (5 alike) : Delay
  cfblk3 : DiscreteIntegrator  SampleTime=-1  OutDataTypeStr=double  ICPrevOutput=DiscIntNeverNeededParam  ICPrevScaledInput=DiscIntNeverNeededParam
  cfblk4 : Delay  ShowEnablePort=on
      settings: InputPortMap=u0,e6
  cfblk5 : If  SampleTime=1
  cfblk8 : Subsystem  TreatAsAtomicUnit=on
  cfblk9 : Subsystem  TreatAsAtomicUnit=on
  cyemi_{641..652,664..666} (15 alike) : DataTypeConversion  OutDataTypeStr=double
  cfblk2 : Outport
  cfblk7 : Outport  Port=2
  wires:
  cfblk3/1 -> cfblk2/1, cyemi_643/1
  cfblk8/1(cfblk2) -> cfblk7/1
  cfblk6/1 -> cyemi_651/1, cyemi_666/1
  cfblk5/1 -> cfblk8/Action
  cfblk5/2 -> cfblk9/Action
  cyemi_641/1 -> cfblk10/1
  cfblk4/1 -> cyemi_641/1
  cyemi_642/1 -> cfblk11/1
  cfblk9/1(cfblk2) -> cyemi_642/1
  cyemi_643/1 -> cfblk12/1
  cyemi_644/1 -> cfblk13/1
  cfblk9/3(cfblk11) -> cyemi_644/1
  cyemi_645/1 -> cfblk14/1
  cfblk9/4(cfblk12) -> cyemi_645/1
  cyemi_646/1 -> cfblk3/1
  cfblk9/2(cfblk10) -> cyemi_646/1
  cyemi_647/1 -> cfblk4/1
  cfblk8/2(cfblk14) -> cyemi_647/1
  cyemi_648/1 -> cfblk4/2
  cfblk13/1 -> cyemi_648/1
  cyemi_649/1 -> cfblk5/1
  cfblk11/1 -> cyemi_649/1
  cyemi_650/1 -> cfblk8/1(cfblk1)
  cfblk1/1 -> cyemi_650/1
  cyemi_651/1 -> cfblk8/2(cfblk12)
  cyemi_652/1 -> cfblk8/3(cfblk13)
  cfblk14/1 -> cyemi_652/1
  cyemi_664/1 -> cfblk9/1(cfblk1)
  cfblk10/1 -> cyemi_664/1
  cyemi_665/1 -> cfblk9/2(cfblk8)
  cfblk12/1 -> cyemi_665/1
  cyemi_666/1 -> cfblk9/3(cfblk9)

== system sampleModel7126_pp/cfblk270 ==
  cfblk1 : Inport
  Action Port : ActionPort  ActionType=else
  cfblk11 : Delay
  cfblk12 : Delay
  cfblk13 : Delay
  cfblk3 : UnitDelay  SampleTime=-1
  cfblk4 : simulink/Discrete/Transfer Fcn Lead or Lag  PoleZ=0.95  ZeroZ=0.75  ICPrevOutput=0.0  ICPrevInput=0.0  DoSatur=off
      settings: SourceProductName=Simulink  SourceProductBaseCode=SL
  cfblk5 : simulink/Continuous/PID Controller (2DOF)  Controller=PID  TimeDomain=Discrete-time  SampleTime=-1  IntegratorMethod=Forward Euler  FilterMethod=Forward Euler  Form=Parallel  UseFilter=on  ControllerParametersSource=internal  P=1  I=1  D=0  N=100  b=1  c=1  InitialConditionSource=internal  InitialConditionForIntegrator=0  InitialConditionForFilter=0  ExternalReset=none  LimitOutput=off  UpperSaturationLimit=inf  LowerSaturationLimit=-inf  LinearizeAsGain=off  AntiWindupMode=none  Kb=1  TrackingMode=off  Kt=1  PParamMin=[]  PParamMax=[]  IParamMin=[]  IParamMax=[]  DParamMin=[]  DParamMax=[]  NParamMin=[]  NParamMax=[]  bParamMin=[]  bParamMax=[]  cParamMin=[]  cParamMax=[]  KbParamMin=[]  KbParamMax=[]  KtParamMin=[]  KtParamMax=[]  POutMin=[]  POutMax=[]  IOutMin=[]  IOutMax=[]  DOutMin=[]  DOutMax=[]  NOutMin=[]  NOutMax=[]  bOutMin=[]  bOutMax=[]  cOutMin=[]  cOutMax=[]  KbOutMin=[]  KbOutMax=[]  KtOutMin=[]  KtOutMax=[]  IntegratorOutMin=[]  IntegratorOutMax=[]  FilterOutMin=[]  FilterOutMax=[]  SumOutMin=[]  SumOutMax=[]  Sum1OutMin=[]  Sum1OutMax=[]  Sum2OutMin=[]  Sum2OutMax=[]  Sum3OutMin=[]  Sum3OutMax=[]  SumI1OutMin=[]  SumI1OutMax=[]  SumI2OutMin=[]  SumI2OutMax=[]  SumI3OutMin=[]  SumI3OutMax=[]  SumDOutMin=[]  SumDOutMax=[]  SaturationOutMin=[]  SaturationOutMax=[]  IntegratorContinuousStateAttributes=''  IntegratorStateMustResolveToSignalObject=off  IntegratorRTWStateStorageClass=Auto  FilterContinuousStateAttributes=''  FilterStateMustResolveToSignalObject=off  FilterRTWStateStorageClass=Auto  DifferentiatorICPrevScaledInput=0  DifferentiatorOutMin=[]  DifferentiatorOutMax=[]  FilterDiffOutCoefMin=[]  FilterDiffOutCoefMax=[]  SumDenOutMin=[]  SumDenOutMax=[]  SumNumOutMin=[]  SumNumOutMax=[]  ReciprocalOutMin=[]  ReciprocalOutMax=[]  DivideOutMin=[]  DivideOutMax=[]  TunerSelectOption=Transfer Function Based (PID Tuner App)
  cfblk6 : simulink/Discrete/Transfer Fcn Lead or Lag  PoleZ=0.95  ZeroZ=0.75  ICPrevOutput=0.0  ICPrevInput=0.0  DoSatur=off
      settings: SourceProductName=Simulink  SourceProductBaseCode=SL
  cfblk7 : simulink/Continuous/PID Controller  Controller=PID  TimeDomain=Discrete-time  SampleTime=-1  IntegratorMethod=Forward Euler  FilterMethod=Forward Euler  Form=Parallel  UseFilter=on  ControllerParametersSource=internal  P=1  I=1  D=0  N=100  InitialConditionSource=internal  InitialConditionForIntegrator=0  InitialConditionForFilter=0  ExternalReset=none  LimitOutput=off  UpperSaturationLimit=inf  LowerSaturationLimit=-inf  LinearizeAsGain=off  AntiWindupMode=none  Kb=1  TrackingMode=off  Kt=1  PParamMin=[]  PParamMax=[]  IParamMin=[]  IParamMax=[]  DParamMin=[]  DParamMax=[]  NParamMin=[]  NParamMax=[]  KbParamMin=[]  KbParamMax=[]  KtParamMin=[]  KtParamMax=[]  POutMin=[]  POutMax=[]  IOutMin=[]  IOutMax=[]  DOutMin=[]  DOutMax=[]  NOutMin=[]  NOutMax=[]  KbOutMin=[]  KbOutMax=[]  KtOutMin=[]  KtOutMax=[]  IntegratorOutMin=[]  IntegratorOutMax=[]  FilterOutMin=[]  FilterOutMax=[]  SumOutMin=[]  SumOutMax=[]  SumI1OutMin=[]  SumI1OutMax=[]  SumI2OutMin=[]  SumI2OutMax=[]  SumI3OutMin=[]  SumI3OutMax=[]  SumDOutMin=[]  SumDOutMax=[]  SaturationOutMin=[]  SaturationOutMax=[]  IntegratorContinuousStateAttributes=''  IntegratorStateMustResolveToSignalObject=off  IntegratorRTWStateStorageClass=Auto  FilterContinuousStateAttributes=''  FilterStateMustResolveToSignalObject=off  FilterRTWStateStorageClass=Auto  DifferentiatorICPrevScaledInput=0  DifferentiatorOutMin=[]  DifferentiatorOutMax=[]  FilterDiffOutCoefMin=[]  FilterDiffOutCoefMax=[]  SumDenOutMin=[]  SumDenOutMax=[]  SumNumOutMin=[]  SumNumOutMax=[]  ReciprocalOutMin=[]  ReciprocalOutMax=[]  DivideOutMin=[]  DivideOutMax=[]  TunerSelectOption=Transfer Function Based (PID Tuner App)
  cfblk8 : Delay  ShowEnablePort=on
      settings: InputPortMap=u0,e6
  cfblk9 : Delay  ShowEnablePort=on
      settings: InputPortMap=u0,e6
  cyemi_{675..687} (13 alike) : DataTypeConversion  OutDataTypeStr=double
  cfblk2 : Outport
  cfblk10 : Outport  Port=2
  wires:
  cfblk5/1 -> cyemi_676/1, cyemi_679/1
  cfblk1/1 -> cfblk2/1, cfblk10/1, cyemi_683/1
  cfblk3/1 -> cyemi_681/1, cyemi_687/1
  cyemi_675/1 -> cfblk11/1
  cfblk4/1 -> cyemi_675/1
  cyemi_676/1 -> cfblk12/1
  cyemi_677/1 -> cfblk13/1
  cfblk6/1 -> cyemi_677/1
  cyemi_678/1 -> cfblk3/1
  cfblk8/1 -> cyemi_678/1
  cyemi_679/1 -> cfblk4/1
  cyemi_680/1 -> cfblk5/1
  cfblk11/1 -> cyemi_680/1
  cyemi_681/1 -> cfblk5/2
  cyemi_682/1 -> cfblk6/1
  cfblk9/1 -> cyemi_682/1
  cyemi_683/1 -> cfblk7/1
  cyemi_684/1 -> cfblk8/1
  cfblk7/1 -> cyemi_684/1
  cyemi_685/1 -> cfblk8/2
  cfblk12/1 -> cyemi_685/1
  cyemi_686/1 -> cfblk9/1
  cfblk13/1 -> cyemi_686/1
  cyemi_687/1 -> cfblk9/2

== system sampleModel7126_pp/cfblk271 ==
  cfblk1 : Inport
  cfblk14 : Inport  Port=2
  Action Port : ActionPort  ActionType=then
  cfblk10 : DiscreteZeroPole  Poles=[0 0.5]  Gain=1  SampleTime=-1
  cfblk11 : simulink/Discrete/Difference  ICPrevInput=0.0  OutMin=[]  OutMax=[]  OutDataTypeStr=double  OutputDataTypeScalingMode=double  OutDataType=fixdt(1, 16)  OutScaling=2^-10  DoSatur=off
  cfblk12 : DiscreteZeroPole  Poles=[0 0.5]  Gain=1  SampleTime=-1
  cfblk13 : simulink/Continuous/PID Controller  Controller=PID  TimeDomain=Discrete-time  SampleTime=-1  IntegratorMethod=Forward Euler  FilterMethod=Forward Euler  Form=Parallel  UseFilter=on  ControllerParametersSource=internal  P=1  I=1  D=0  N=100  InitialConditionSource=internal  InitialConditionForIntegrator=0  InitialConditionForFilter=0  ExternalReset=none  LimitOutput=off  UpperSaturationLimit=inf  LowerSaturationLimit=-inf  LinearizeAsGain=off  AntiWindupMode=none  Kb=1  TrackingMode=off  Kt=1  PParamMin=[]  PParamMax=[]  IParamMin=[]  IParamMax=[]  DParamMin=[]  DParamMax=[]  NParamMin=[]  NParamMax=[]  KbParamMin=[]  KbParamMax=[]  KtParamMin=[]  KtParamMax=[]  POutMin=[]  POutMax=[]  IOutMin=[]  IOutMax=[]  DOutMin=[]  DOutMax=[]  NOutMin=[]  NOutMax=[]  KbOutMin=[]  KbOutMax=[]  KtOutMin=[]  KtOutMax=[]  IntegratorOutMin=[]  IntegratorOutMax=[]  FilterOutMin=[]  FilterOutMax=[]  SumOutMin=[]  SumOutMax=[]  SumI1OutMin=[]  SumI1OutMax=[]  SumI2OutMin=[]  SumI2OutMax=[]  SumI3OutMin=[]  SumI3OutMax=[]  SumDOutMin=[]  SumDOutMax=[]  SaturationOutMin=[]  SaturationOutMax=[]  IntegratorContinuousStateAttributes=''  IntegratorStateMustResolveToSignalObject=off  IntegratorRTWStateStorageClass=Auto  FilterContinuousStateAttributes=''  FilterStateMustResolveToSignalObject=off  FilterRTWStateStorageClass=Auto  DifferentiatorICPrevScaledInput=0  DifferentiatorOutMin=[]  DifferentiatorOutMax=[]  FilterDiffOutCoefMin=[]  FilterDiffOutCoefMax=[]  SumDenOutMin=[]  SumDenOutMax=[]  SumNumOutMin=[]  SumNumOutMax=[]  ReciprocalOutMin=[]  ReciprocalOutMax=[]  DivideOutMin=[]  DivideOutMax=[]  TunerSelectOption=Transfer Function Based (PID Tuner App)
  cfblk15 : Delay
  cfblk16 : Delay
  cfblk3 : UnitDelay  SampleTime=-1
  cfblk4 : Delay  DelayLengthSource=Input port
      settings: InputPortMap=u0,p1
  cfblk5 : simulink/Discrete/Difference  ICPrevInput=0.0  OutMin=[]  OutMax=[]  OutDataTypeStr=double  OutputDataTypeScalingMode=double  OutDataType=fixdt(1, 16)  OutScaling=2^-10  DoSatur=off
  cfblk6 : Delay  DelayLengthSource=Input port
      settings: InputPortMap=u0,p1
  cfblk7 : simulink/Continuous/PID Controller (2DOF)  Controller=PID  TimeDomain=Discrete-time  SampleTime=-1  IntegratorMethod=Forward Euler  FilterMethod=Forward Euler  Form=Parallel  UseFilter=on  ControllerParametersSource=internal  P=1  I=1  D=0  N=100  b=1  c=1  InitialConditionSource=internal  InitialConditionForIntegrator=0  InitialConditionForFilter=0  ExternalReset=none  LimitOutput=off  UpperSaturationLimit=inf  LowerSaturationLimit=-inf  LinearizeAsGain=off  AntiWindupMode=none  Kb=1  TrackingMode=off  Kt=1  PParamMin=[]  PParamMax=[]  IParamMin=[]  IParamMax=[]  DParamMin=[]  DParamMax=[]  NParamMin=[]  NParamMax=[]  bParamMin=[]  bParamMax=[]  cParamMin=[]  cParamMax=[]  KbParamMin=[]  KbParamMax=[]  KtParamMin=[]  KtParamMax=[]  POutMin=[]  POutMax=[]  IOutMin=[]  IOutMax=[]  DOutMin=[]  DOutMax=[]  NOutMin=[]  NOutMax=[]  bOutMin=[]  bOutMax=[]  cOutMin=[]  cOutMax=[]  KbOutMin=[]  KbOutMax=[]  KtOutMin=[]  KtOutMax=[]  IntegratorOutMin=[]  IntegratorOutMax=[]  FilterOutMin=[]  FilterOutMax=[]  SumOutMin=[]  SumOutMax=[]  Sum1OutMin=[]  Sum1OutMax=[]  Sum2OutMin=[]  Sum2OutMax=[]  Sum3OutMin=[]  Sum3OutMax=[]  SumI1OutMin=[]  SumI1OutMax=[]  SumI2OutMin=[]  SumI2OutMax=[]  SumI3OutMin=[]  SumI3OutMax=[]  SumDOutMin=[]  SumDOutMax=[]  SaturationOutMin=[]  SaturationOutMax=[]  IntegratorContinuousStateAttributes=''  IntegratorStateMustResolveToSignalObject=off  IntegratorRTWStateStorageClass=Auto  FilterContinuousStateAttributes=''  FilterStateMustResolveToSignalObject=off  FilterRTWStateStorageClass=Auto  DifferentiatorICPrevScaledInput=0  DifferentiatorOutMin=[]  DifferentiatorOutMax=[]  FilterDiffOutCoefMin=[]  FilterDiffOutCoefMax=[]  SumDenOutMin=[]  SumDenOutMax=[]  SumNumOutMin=[]  SumNumOutMax=[]  ReciprocalOutMin=[]  ReciprocalOutMax=[]  DivideOutMin=[]  DivideOutMax=[]  TunerSelectOption=Transfer Function Based (PID Tuner App)
  cfblk8 : UnitDelay  SampleTime=-1
  cfblk9 : simulink/Discrete/Transfer Fcn Real Zero  ZeroZ=0.75  ICPrevInput=0.0  DoSatur=off
      settings: SourceProductName=Simulink  SourceProductBaseCode=SL
  cyemi_{690..705} (16 alike) : DataTypeConversion  OutDataTypeStr=double
  cfblk2 : Outport
  wires:
  cfblk13/1 -> cfblk2/1
  cfblk3/1 -> cyemi_693/1, cyemi_703/1
  cfblk9/1 -> cyemi_690/1, cyemi_695/1
  cyemi_690/1 -> cfblk10/1
  cyemi_691/1 -> cfblk11/1
  cfblk14/1 -> cyemi_691/1
  cyemi_692/1 -> cfblk12/1
  cfblk1/1 -> cyemi_692/1
  cyemi_693/1 -> cfblk13/1
  cyemi_694/1 -> cfblk15/1
  cfblk5/1 -> cyemi_694/1
  cyemi_695/1 -> cfblk16/1
  cyemi_696/1 -> cfblk3/1
  cfblk6/1 -> cyemi_696/1
  cyemi_697/1 -> cfblk4/1
  cfblk8/1 -> cyemi_697/1
  cyemi_698/1 -> cfblk4/2
  cfblk16/1 -> cyemi_698/1
  cyemi_699/1 -> cfblk5/1
  cfblk10/1 -> cyemi_699/1
  cyemi_700/1 -> cfblk6/1
  cfblk15/1 -> cyemi_700/1
  cyemi_701/1 -> cfblk6/2
  cfblk12/1 -> cyemi_701/1
  cyemi_702/1 -> cfblk7/1
  cfblk11/1 -> cyemi_702/1
  cyemi_703/1 -> cfblk7/2
  cyemi_704/1 -> cfblk8/1
  cfblk7/1 -> cyemi_704/1
  cyemi_705/1 -> cfblk9/1
  cfblk4/1 -> cyemi_705/1

== system sampleModel7126_pp/cfblk272 ==
  cfblk1 : Inport
  cfblk9 : Inport  Port=2
  Action Port : ActionPort  ActionType=else
  cfblk11 : Delay
  cfblk12 : DataTypeConversion  OutDataTypeStr=double
  cfblk13 : DataTypeConversion  OutDataTypeStr=double
  cfblk3 : Delay  ShowEnablePort=on
      settings: InputPortMap=u0,e6
  cfblk4 : DiscreteIntegrator  SampleTime=-1  OutDataTypeStr=double  ICPrevOutput=DiscIntNeverNeededParam  ICPrevScaledInput=DiscIntNeverNeededParam
  cfblk5 : simulink/Continuous/PID Controller (2DOF)  Controller=PID  TimeDomain=Discrete-time  SampleTime=-1  IntegratorMethod=Forward Euler  FilterMethod=Forward Euler  Form=Parallel  UseFilter=on  ControllerParametersSource=internal  P=1  I=1  D=0  N=100  b=1  c=1  InitialConditionSource=internal  InitialConditionForIntegrator=0  InitialConditionForFilter=0  ExternalReset=none  LimitOutput=off  UpperSaturationLimit=inf  LowerSaturationLimit=-inf  LinearizeAsGain=off  AntiWindupMode=none  Kb=1  TrackingMode=off  Kt=1  PParamMin=[]  PParamMax=[]  IParamMin=[]  IParamMax=[]  DParamMin=[]  DParamMax=[]  NParamMin=[]  NParamMax=[]  bParamMin=[]  bParamMax=[]  cParamMin=[]  cParamMax=[]  KbParamMin=[]  KbParamMax=[]  KtParamMin=[]  KtParamMax=[]  POutMin=[]  POutMax=[]  IOutMin=[]  IOutMax=[]  DOutMin=[]  DOutMax=[]  NOutMin=[]  NOutMax=[]  bOutMin=[]  bOutMax=[]  cOutMin=[]  cOutMax=[]  KbOutMin=[]  KbOutMax=[]  KtOutMin=[]  KtOutMax=[]  IntegratorOutMin=[]  IntegratorOutMax=[]  FilterOutMin=[]  FilterOutMax=[]  SumOutMin=[]  SumOutMax=[]  Sum1OutMin=[]  Sum1OutMax=[]  Sum2OutMin=[]  Sum2OutMax=[]  Sum3OutMin=[]  Sum3OutMax=[]  SumI1OutMin=[]  SumI1OutMax=[]  SumI2OutMin=[]  SumI2OutMax=[]  SumI3OutMin=[]  SumI3OutMax=[]  SumDOutMin=[]  SumDOutMax=[]  SaturationOutMin=[]  SaturationOutMax=[]  IntegratorContinuousStateAttributes=''  IntegratorStateMustResolveToSignalObject=off  IntegratorRTWStateStorageClass=Auto  FilterContinuousStateAttributes=''  FilterStateMustResolveToSignalObject=off  FilterRTWStateStorageClass=Auto  DifferentiatorICPrevScaledInput=0  DifferentiatorOutMin=[]  DifferentiatorOutMax=[]  FilterDiffOutCoefMin=[]  FilterDiffOutCoefMax=[]  SumDenOutMin=[]  SumDenOutMax=[]  SumNumOutMin=[]  SumNumOutMax=[]  ReciprocalOutMin=[]  ReciprocalOutMax=[]  DivideOutMin=[]  DivideOutMax=[]  TunerSelectOption=Transfer Function Based (PID Tuner App)
  cfblk6 : UnitDelay  SampleTime=-1
  cfblk7 : DiscreteTransferFcn
  cfblk8 : UnitDelay  SampleTime=-1
  cyemi_{708..709,711..718} (10 alike) : DataTypeConversion  OutDataTypeStr=double
  cyemi_710 : DataTypeConversion  OutDataTypeStr=uint16
  cfblk2 : Outport
  cfblk10 : Outport  Port=2
  wires:
  cfblk6/1 -> cfblk2/1
  cfblk3/1 -> cyemi_713/1, cyemi_718/1
  cfblk4/1 -> cfblk10/1
  cfblk1/1 -> cyemi_712/1, cyemi_715/1
  cyemi_708/1 -> cfblk11/1
  cfblk5/1 -> cyemi_708/1
  cyemi_709/1 -> cfblk12/1
  cfblk7/1 -> cyemi_709/1
  cyemi_710/1 -> cfblk13/1
  cfblk9/1 -> cyemi_710/1
  cyemi_711/1 -> cfblk3/1
  cfblk11/1 -> cyemi_711/1
  cyemi_712/1 -> cfblk3/2
  cyemi_713/1 -> cfblk4/1
  cyemi_714/1 -> cfblk5/1
  cfblk8/1 -> cyemi_714/1
  cyemi_715/1 -> cfblk5/2
  cyemi_716/1 -> cfblk6/1
  cfblk12/1 -> cyemi_716/1
  cyemi_717/1 -> cfblk7/1
  cfblk13/1 -> cyemi_717/1
  cyemi_718/1 -> cfblk8/1

== system sampleModel7126_pp/cfblk273 ==
  cfblk1 : Inport
  cfblk8 : Inport  Port=2
  Action Port : ActionPort  ActionType=then
  cfblk10 : Subsystem  TreatAsAtomicUnit=on
  cfblk11 : Delay
  cfblk12 : Delay
  cfblk3 : simulink/Discrete/Tapped Delay  vinit=0.0  samptime=-1  NumDelays=1  DelayOrder=Oldest  includeCurrent=off
  cfblk4 : UnitDelay  SampleTime=-1
  cfblk5 : DiscreteZeroPole  Poles=[0 0.5]  Gain=1  SampleTime=-1
  cfblk6 : DiscreteZeroPole  Poles=[0 0.5]  Gain=1  SampleTime=-1
  cfblk7 : If  SampleTime=1
  cfblk9 : Subsystem  TreatAsAtomicUnit=on
  cyemi_{721..722,733..742} (12 alike) : DataTypeConversion  OutDataTypeStr=double
  cfblk2 : Outport
  wires:
  cfblk3/1 -> cyemi_738/1, cyemi_742/1
  cfblk9/1(cfblk2) -> cfblk2/1
  cfblk7/1 -> cfblk9/Action
  cfblk7/2 -> cfblk10/Action
  cyemi_721/1 -> cfblk10/1(cfblk1)
  cfblk4/1 -> cyemi_721/1
  cyemi_722/1 -> cfblk10/2(cfblk12)
  cfblk6/1 -> cyemi_722/1
  cyemi_733/1 -> cfblk11/1
  cfblk9/2(cfblk13) -> cyemi_733/1
  cyemi_734/1 -> cfblk12/1
  cfblk5/1 -> cyemi_734/1
  cyemi_735/1 -> cfblk3/1
  cfblk1/1 -> cyemi_735/1
  cyemi_736/1 -> cfblk4/1
  cfblk8/1 -> cyemi_736/1
  cyemi_737/1 -> cfblk5/1
  cfblk10/2(cfblk13) -> cyemi_737/1
  cyemi_738/1 -> cfblk6/1
  cyemi_739/1 -> cfblk7/1
  cfblk11/1 -> cyemi_739/1
  cyemi_740/1 -> cfblk9/1(cfblk1)
  cfblk10/1(cfblk2) -> cyemi_740/1
  cyemi_741/1 -> cfblk9/2(cfblk11)
  cfblk12/1 -> cyemi_741/1
  cyemi_742/1 -> cfblk9/3(cfblk12)

== system sampleModel7126_pp/cfblk274 ==
  cfblk1 : Inport
  Action Port : ActionPort  ActionType=else
  cfblk10 : Delay
  cfblk3 : DiscreteTransferFcn
  cfblk4 : DiscreteIntegrator  SampleTime=-1  OutDataTypeStr=double  ICPrevOutput=DiscIntNeverNeededParam  ICPrevScaledInput=DiscIntNeverNeededParam
  cfblk5 : DiscreteTransferFcn
  cfblk6 : Delay  ShowEnablePort=on
      settings: InputPortMap=u0,e6
  cfblk7 : Delay  ShowEnablePort=on
      settings: InputPortMap=u0,e6
  cfblk9 : Delay
  cyemi_{754..762} (9 alike) : DataTypeConversion  OutDataTypeStr=double
  cfblk2 : Outport
  cfblk8 : Outport  Port=2
  wires:
  cfblk5/1 -> cyemi_754/1, cyemi_762/1
  cfblk1/1 -> cfblk2/1
  cfblk7/1 -> cfblk8/1, cyemi_756/1
  cyemi_754/1 -> cfblk10/1
  cyemi_755/1 -> cfblk3/1
  cfblk10/1 -> cyemi_755/1
  cyemi_756/1 -> cfblk4/1
  cyemi_757/1 -> cfblk5/1
  cfblk4/1 -> cyemi_757/1
  cyemi_758/1 -> cfblk6/1
  cfblk9/1 -> cyemi_758/1
  cyemi_759/1 -> cfblk6/2
  cfblk3/1 -> cyemi_759/1
  cyemi_760/1 -> cfblk7/1
  cfblk6/1 -> cyemi_760/1, cyemi_761/1
  cyemi_761/1 -> cfblk7/2
  cyemi_762/1 -> cfblk9/1
